simulink model "STM32_UART_Receiver2_2016b"  (R2016b)
settings: Solver=FixedStepDiscrete  StartTime=0.0  StopTime=inf  FixedStep=0.02  RelTol=1e-3  EnableMultiTasking=on
undefined symbols (not defined in the file or in its folder): serial
libraries: xpcutilitieslib x25, etargetslib x25, instrumentlib x2, aerolibanimutils x1
settings Model: Creator=Administrator  LastModifiedBy=Administrator
settings DataIOCC: LimitDataPoints=on  SaveFormat=Array
settings OptimizationCC: LifeSpan=inf
settings DebuggingCC: SFUnexpectedBacktrackingDiag=warning  SFNoUnconditionalDefaultTransitionDiag=warning  SFExecutionAtInitializationDiag=none
settings HardwareCC: ProdBitPerPointer=32  ProdBitPerSizeT=32  ProdBitPerPtrDiffT=32  ProdLargestAtomicFloat=None  ProdIntDivRoundTo=Undefined  ProdEndianess=Unspecified  ProdWordSize=32  ProdHWDeviceType=32-bit Generic
settings ModelReferenceCC: PropagateSignalLabelsOutOfModel=off
settings GRTTargetCC: TargetLangStandard=C89/C90 (ANSI)  GeneratePreprocessorConditionals=Disable all
settings ConfigComp: CovMetricSettings=dw  CovHtmlReporting=on  CovSaveCumulativeToWorkspaceVar=on  CovSaveSingleToWorkspaceVar=on  CovExternalEMLEnable=off

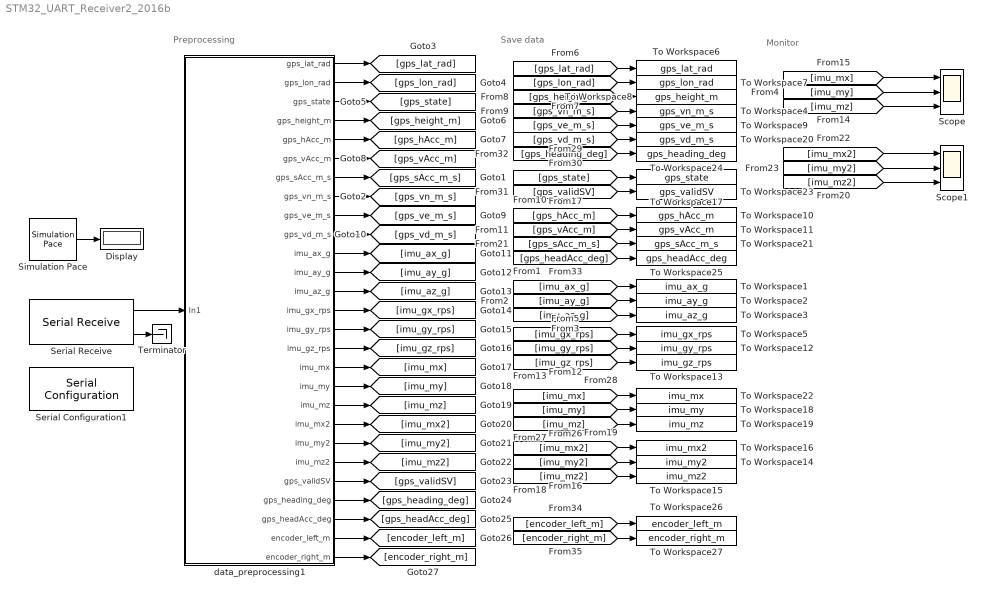
== system STM32_UART_Receiver2_2016b ==
  note: Monitor
  note: Preprocessing
  note: Save data
  Display : Display
  Scope : Scope  NumInputPorts=3
  Scope1 : Scope  NumInputPorts=3
  Serial Configuration1 : instrumentlib/Serial Configuration  Priority=-200000  ComPortMenu=<Please select a port...>  ComPort=COM8  ObjConstructor=serial('COM8');  BaudRate=9600  DataBits=8  Parity=none  StopBits=1  FlowControl=none  Timeout=10  ByteOrder=LittleEndian
  Serial Receive : instrumentlib/Serial Receive  ComPortMenu=<Please select a port...>  ComPort=COM8  ObjConstructor=serial('COM8');  Header=AA1  Terminator=<none>  DataSize="[1  72]"  DataType=uint8  EnableBlockingMode=off  ActionDataUnavailable=Output last received value  CustomValue=0  SampleTime=0.02
  Simulation Pace : aerolibanimutils/Simulation Pace  SimulationPace=1  SleepMode=MATLAB Thread  OutputPaceError=on  SampleTime=0.02
  Terminator : Terminator
  To Workspace1 : ToWorkspace  VariableName=imu_ax_g  SampleTime=-1
      settings: Save2DSignal=2-D array (concatenate along first dimension)
  To Workspace10 : ToWorkspace  VariableName=gps_hAcc_m  SampleTime=-1
      settings: Save2DSignal=2-D array (concatenate along first dimension)
  To Workspace11 : ToWorkspace  VariableName=gps_vAcc_m  SampleTime=-1
      settings: Save2DSignal=2-D array (concatenate along first dimension)
  To Workspace12 : ToWorkspace  VariableName=imu_gy_rps  SampleTime=-1
      settings: Save2DSignal=2-D array (concatenate along first dimension)
  To Workspace13 : ToWorkspace  VariableName=imu_gz_rps  SampleTime=-1
      settings: Save2DSignal=2-D array (concatenate along first dimension)
  To Workspace14 : ToWorkspace  VariableName=imu_my2  SampleTime=-1
      settings: Save2DSignal=2-D array (concatenate along first dimension)
  To Workspace15 : ToWorkspace  VariableName=imu_mz2  SampleTime=-1
      settings: Save2DSignal=2-D array (concatenate along first dimension)
  To Workspace16 : ToWorkspace  VariableName=imu_mx2  SampleTime=-1
      settings: Save2DSignal=2-D array (concatenate along first dimension)
  To Workspace17 : ToWorkspace  VariableName=gps_state  SampleTime=-1
      settings: Save2DSignal=2-D array (concatenate along first dimension)
  To Workspace18 : ToWorkspace  VariableName=imu_my  SampleTime=-1
      settings: Save2DSignal=2-D array (concatenate along first dimension)
  To Workspace19 : ToWorkspace  VariableName=imu_mz  SampleTime=-1
      settings: Save2DSignal=2-D array (concatenate along first dimension)
  To Workspace2 : ToWorkspace  VariableName=imu_ay_g  SampleTime=-1
      settings: Save2DSignal=2-D array (concatenate along first dimension)
  To Workspace20 : ToWorkspace  VariableName=gps_vd_m_s  SampleTime=-1
      settings: Save2DSignal=2-D array (concatenate along first dimension)
  To Workspace21 : ToWorkspace  VariableName=gps_sAcc_m_s  SampleTime=-1
      settings: Save2DSignal=2-D array (concatenate along first dimension)
  To Workspace22 : ToWorkspace  VariableName=imu_mx  SampleTime=-1
      settings: Save2DSignal=2-D array (concatenate along first dimension)
  To Workspace23 : ToWorkspace  VariableName=gps_validSV  SampleTime=-1
      settings: Save2DSignal=2-D array (concatenate along first dimension)
  To Workspace24 : ToWorkspace  VariableName=gps_heading_deg  SampleTime=-1
      settings: Save2DSignal=2-D array (concatenate along first dimension)
  To Workspace25 : ToWorkspace  VariableName=gps_headAcc_deg  SampleTime=-1
      settings: Save2DSignal=2-D array (concatenate along first dimension)
  To Workspace26 : ToWorkspace  VariableName=encoder_left_m  SampleTime=-1
      settings: Save2DSignal=2-D array (concatenate along first dimension)
  To Workspace27 : ToWorkspace  VariableName=encoder_right_m  SampleTime=-1
      settings: Save2DSignal=2-D array (concatenate along first dimension)
  To Workspace3 : ToWorkspace  VariableName=imu_az_g  SampleTime=-1
      settings: Save2DSignal=2-D array (concatenate along first dimension)
  To Workspace4 : ToWorkspace  VariableName=gps_vn_m_s  SampleTime=-1
      settings: Save2DSignal=2-D array (concatenate along first dimension)
  To Workspace5 : ToWorkspace  VariableName=imu_gx_rps  SampleTime=-1
      settings: Save2DSignal=2-D array (concatenate along first dimension)
  To Workspace6 : ToWorkspace  VariableName=gps_lat_rad  SampleTime=-1
      settings: Save2DSignal=2-D array (concatenate along first dimension)
  To Workspace7 : ToWorkspace  VariableName=gps_lon_rad  SampleTime=-1
      settings: Save2DSignal=2-D array (concatenate along first dimension)
  To Workspace8 : ToWorkspace  VariableName=gps_height_m  SampleTime=-1
      settings: Save2DSignal=2-D array (concatenate along first dimension)
  To Workspace9 : ToWorkspace  VariableName=gps_ve_m_s  SampleTime=-1
      settings: Save2DSignal=2-D array (concatenate along first dimension)
  data_preprocessing1 : Subsystem
  wires:
  [gps_lat_rad] -> To Workspace6/1
  [gps_lon_rad] -> To Workspace7/1
  [gps_height_m] -> To Workspace8/1
  [gps_hAcc_m] -> To Workspace10/1
  [gps_vAcc_m] -> To Workspace11/1
  [gps_sAcc_m_s] -> To Workspace21/1
  [imu_ax_g] -> To Workspace1/1
  [imu_ay_g] -> To Workspace2/1
  [imu_az_g] -> To Workspace3/1
  [imu_gx_rps] -> To Workspace5/1
  [imu_gy_rps] -> To Workspace12/1
  [imu_gz_rps] -> To Workspace13/1
  data_preprocessing1/1(gps_lat_rad) -> [gps_lat_rad]
  data_preprocessing1/2(gps_lon_rad) -> [gps_lon_rad]
  data_preprocessing1/3(gps_state) -> [gps_state]
  data_preprocessing1/4(gps_height_m) -> [gps_height_m]
  data_preprocessing1/5(gps_hAcc_m) -> [gps_hAcc_m]
  data_preprocessing1/6(gps_vAcc_m) -> [gps_vAcc_m]
  data_preprocessing1/7(gps_sAcc_m_s) -> [gps_sAcc_m_s]
  data_preprocessing1/8(gps_vn_m_s) -> [gps_vn_m_s]
  data_preprocessing1/9(gps_ve_m_s) -> [gps_ve_m_s]
  data_preprocessing1/10(gps_vd_m_s) -> [gps_vd_m_s]
  data_preprocessing1/11(imu_ax_g) -> [imu_ax_g]
  data_preprocessing1/12(imu_ay_g) -> [imu_ay_g]
  data_preprocessing1/13(imu_az_g) -> [imu_az_g]
  data_preprocessing1/14(imu_gx_rps) -> [imu_gx_rps]
  data_preprocessing1/15(imu_gy_rps) -> [imu_gy_rps]
  data_preprocessing1/16(imu_gz_rps) -> [imu_gz_rps]
  data_preprocessing1/17(imu_mx) -> [imu_mx]
  data_preprocessing1/19(imu_mz) -> [imu_mz]
  [imu_mx] -> To Workspace22/1
  [imu_my] -> To Workspace18/1
  [imu_mz] -> To Workspace19/1
  [gps_state] -> To Workspace17/1
  [gps_vn_m_s] -> To Workspace4/1
  [gps_ve_m_s] -> To Workspace9/1
  [gps_vd_m_s] -> To Workspace20/1
  data_preprocessing1/18(imu_my) -> [imu_my]
  data_preprocessing1/23(gps_validSV) -> [gps_validSV]
  data_preprocessing1/24(gps_heading_deg) -> [gps_heading_deg]
  data_preprocessing1/25(gps_headAcc_deg) -> [gps_headAcc_deg]
  [gps_heading_deg] -> To Workspace24/1
  [gps_headAcc_deg] -> To Workspace25/1
  [gps_validSV] -> To Workspace23/1
  data_preprocessing1/26(encoder_left_m) -> [encoder_left_m]
  data_preprocessing1/27(encoder_right_m) -> [encoder_right_m]
  [encoder_left_m] -> To Workspace26/1
  [encoder_right_m] -> To Workspace27/1
  Serial Receive/1 -> data_preprocessing1/1(In1)
  Simulation Pace/1 -> Display/1
  [imu_mx] -> Scope/1
  [imu_my] -> Scope/2
  [imu_mz] -> Scope/3
  data_preprocessing1/20(imu_mx2) -> [imu_mx2]
  data_preprocessing1/21(imu_my2) -> [imu_my2]
  data_preprocessing1/22(imu_mz2) -> [imu_mz2]
  [imu_mx2] -> To Workspace16/1
  [imu_my2] -> To Workspace14/1
  [imu_mz2] -> To Workspace15/1
  [imu_mx2] -> Scope1/1
  [imu_my2] -> Scope1/2
  [imu_mz2] -> Scope1/3
  Serial Receive/2 -> Terminator/1

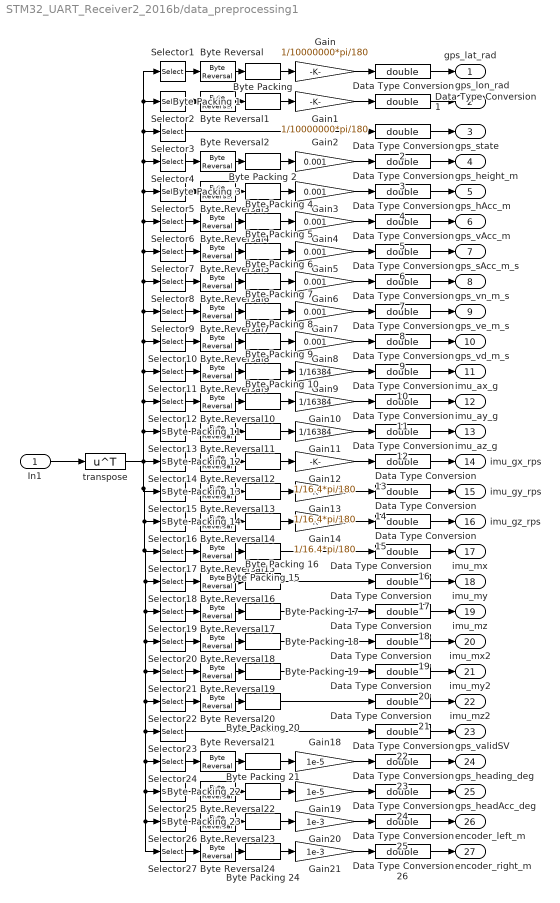
== system STM32_UART_Receiver2_2016b/data_preprocessing1 ==
  In1 : Inport
  Byte Packing {,1..24} (25 alike) : xpcutilitieslib/Byte Packing 
  Byte Reversal{,1..24} (25 alike) : etargetslib/Byte Reversal  numInp=1
  Data Type Conversion{,1..26} (27 alike) : DataTypeConversion  OutDataTypeStr=double
  Gain : Gain  Gain=1/10000000*pi/180
  Gain1 : Gain  Gain=1/10000000*pi/180
  Gain10 : Gain  Gain=1/16384
  Gain11 : Gain  Gain=1/16384
  Gain12 : Gain  Gain=1/16.4*pi/180
  Gain13 : Gain  Gain=1/16.4*pi/180
  Gain14 : Gain  Gain=1/16.4*pi/180
  Gain18 : Gain  Gain=1e-5
  Gain19 : Gain  Gain=1e-5
  Gain{2..8} (7 alike) : Gain  Gain=0.001
  Gain20 : Gain  Gain=1e-3
  Gain21 : Gain  Gain=1e-3
  Gain9 : Gain  Gain=1/16384
  Selector1 : Selector  InputPortWidth=72  IndexOptions=Index vector (dialog)  Indices=[5 4 3 2]  OutputSizes=1
  Selector10 : Selector  InputPortWidth=72  IndexOptions=Index vector (dialog)  Indices=[32 31 30 29]  OutputSizes=1
  Selector11 : Selector  InputPortWidth=72  IndexOptions=Index vector (dialog)  Indices=[34 33]  OutputSizes=1
  Selector12 : Selector  InputPortWidth=72  IndexOptions=Index vector (dialog)  Indices=[36 35]  OutputSizes=1
  Selector13 : Selector  InputPortWidth=72  IndexOptions=Index vector (dialog)  Indices=[38 37]  OutputSizes=1
  Selector14 : Selector  InputPortWidth=72  IndexOptions=Index vector (dialog)  Indices=[40 39]  OutputSizes=1
  Selector15 : Selector  InputPortWidth=72  IndexOptions=Index vector (dialog)  Indices=[42 41]  OutputSizes=1
  Selector16 : Selector  InputPortWidth=72  IndexOptions=Index vector (dialog)  Indices=[44 43]  OutputSizes=1
  Selector17 : Selector  InputPortWidth=72  IndexOptions=Index vector (dialog)  Indices=[46 45]  OutputSizes=1
  Selector18 : Selector  InputPortWidth=72  IndexOptions=Index vector (dialog)  Indices=[48 47]  OutputSizes=1
  Selector19 : Selector  InputPortWidth=72  IndexOptions=Index vector (dialog)  Indices=[50 49]  OutputSizes=1
  Selector2 : Selector  InputPortWidth=72  IndexOptions=Index vector (dialog)  Indices=[9 8 7 6]  OutputSizes=1
  Selector20 : Selector  InputPortWidth=72  IndexOptions=Index vector (dialog)  Indices=[52 51]  OutputSizes=1
  Selector21 : Selector  InputPortWidth=72  IndexOptions=Index vector (dialog)  Indices=[54 53]  OutputSizes=1
  Selector22 : Selector  InputPortWidth=72  IndexOptions=Index vector (dialog)  Indices=[56 55]  OutputSizes=1
  Selector23 : Selector  InputPortWidth=72  IndexOptions=Index vector (dialog)  Indices=57  OutputSizes=1
  Selector24 : Selector  InputPortWidth=72  IndexOptions=Index vector (dialog)  Indices=[61 60 59 58]  OutputSizes=1
  Selector25 : Selector  InputPortWidth=72  IndexOptions=Index vector (dialog)  Indices=[63 62]  OutputSizes=1
  Selector26 : Selector  InputPortWidth=72  IndexOptions=Index vector (dialog)  Indices=[67 66 65 64]  OutputSizes=1
  Selector27 : Selector  InputPortWidth=72  IndexOptions=Index vector (dialog)  Indices=[71 70 69 68]  OutputSizes=1
  Selector3 : Selector  InputPortWidth=72  IndexOptions=Index vector (dialog)  Indices=10  OutputSizes=1
  Selector4 : Selector  InputPortWidth=72  IndexOptions=Index vector (dialog)  Indices=[14 13 12 11]  OutputSizes=1
  Selector5 : Selector  InputPortWidth=72  IndexOptions=Index vector (dialog)  Indices=[16 15]  OutputSizes=1
  Selector6 : Selector  InputPortWidth=72  IndexOptions=Index vector (dialog)  Indices=[18 17]  OutputSizes=1
  Selector7 : Selector  InputPortWidth=72  IndexOptions=Index vector (dialog)  Indices=[20 19]  OutputSizes=1
  Selector8 : Selector  InputPortWidth=72  IndexOptions=Index vector (dialog)  Indices=[24 23 22 21]  OutputSizes=1
  Selector9 : Selector  InputPortWidth=72  IndexOptions=Index vector (dialog)  Indices=[28 27 26 25]  OutputSizes=1
  transpose : Math  Operator=transpose  SaturateOnIntegerOverflow=on
  gps_lat_rad : Outport
  gps_lon_rad : Outport  Port=2
  gps_state : Outport  Port=3
  gps_height_m : Outport  Port=4
  gps_hAcc_m : Outport  Port=5
  gps_vAcc_m : Outport  Port=6
  gps_sAcc_m_s : Outport  Port=7
  gps_vn_m_s : Outport  Port=8
  gps_ve_m_s : Outport  Port=9
  gps_vd_m_s : Outport  Port=10
  imu_ax_g : Outport  Port=11
  imu_ay_g : Outport  Port=12
  imu_az_g : Outport  Port=13
  imu_gx_rps : Outport  Port=14
  imu_gy_rps : Outport  Port=15
  imu_gz_rps : Outport  Port=16
  imu_mx : Outport  Port=17
  imu_my : Outport  Port=18
  imu_mz : Outport  Port=19
  imu_mx2 : Outport  Port=20
  imu_my2 : Outport  Port=21
  imu_mz2 : Outport  Port=22
  gps_validSV : Outport  Port=23
  gps_heading_deg : Outport  Port=24
  gps_headAcc_deg : Outport  Port=25
  encoder_left_m : Outport  Port=26
  encoder_right_m : Outport  Port=27
  wires:
  In1/1 -> transpose/1
  Gain/1 -> Data Type Conversion/1
  "Byte Packing "/1 -> Gain/1
  Selector1/1 -> Byte Reversal/1
  Byte Reversal/1 -> "Byte Packing "/1
  Selector2/1 -> Byte Reversal1/1
  Byte Reversal1/1 -> Byte Packing 1/1
  Byte Packing 1/1 -> Gain1/1
  Gain1/1 -> Data Type Conversion1/1
  Selector3/1 -> Data Type Conversion2/1
  Byte Packing 2/1 -> Gain2/1
  Byte Reversal2/1 -> Byte Packing 2/1
  Selector4/1 -> Byte Reversal2/1
  Gain2/1 -> Data Type Conversion3/1
  Selector5/1 -> Byte Reversal3/1
  Byte Reversal3/1 -> Byte Packing 3/1
  Byte Packing 3/1 -> Gain3/1
  Gain3/1 -> Data Type Conversion4/1
  Selector6/1 -> Byte Reversal4/1
  Byte Reversal4/1 -> Byte Packing 4/1
  Byte Packing 4/1 -> Gain4/1
  Gain4/1 -> Data Type Conversion5/1
  Byte Packing 5/1 -> Gain5/1
  Selector7/1 -> Byte Reversal5/1
  Byte Reversal5/1 -> Byte Packing 5/1
  Gain5/1 -> Data Type Conversion6/1
  Byte Packing 6/1 -> Gain6/1
  Byte Reversal6/1 -> Byte Packing 6/1
  Selector8/1 -> Byte Reversal6/1
  Gain6/1 -> Data Type Conversion7/1
  Byte Reversal7/1 -> Byte Packing 7/1
  Selector9/1 -> Byte Reversal7/1
  Byte Packing 7/1 -> Gain7/1
  Gain7/1 -> Data Type Conversion8/1
  Byte Reversal8/1 -> Byte Packing 8/1
  Selector10/1 -> Byte Reversal8/1
  Byte Packing 8/1 -> Gain8/1
  Gain8/1 -> Data Type Conversion9/1
  Selector11/1 -> Byte Reversal9/1
  Byte Reversal9/1 -> Byte Packing 9/1
  Gain9/1 -> Data Type Conversion10/1
  Byte Packing 9/1 -> Gain9/1
  Byte Reversal10/1 -> Byte Packing 10/1
  Byte Packing 10/1 -> Gain10/1
  Selector12/1 -> Byte Reversal10/1
  Gain10/1 -> Data Type Conversion11/1
  Byte Reversal11/1 -> Byte Packing 11/1
  Selector13/1 -> Byte Reversal11/1
  Byte Packing 11/1 -> Gain11/1
  Gain11/1 -> Data Type Conversion12/1
  Byte Reversal12/1 -> Byte Packing 12/1
  Byte Packing 12/1 -> Gain12/1
  Selector14/1 -> Byte Reversal12/1
  Gain12/1 -> Data Type Conversion13/1
  Byte Packing 13/1 -> Gain13/1
  Byte Reversal13/1 -> Byte Packing 13/1
  Selector15/1 -> Byte Reversal13/1
  Gain13/1 -> Data Type Conversion14/1
  Byte Packing 14/1 -> Gain14/1
  Byte Reversal14/1 -> Byte Packing 14/1
  Selector16/1 -> Byte Reversal14/1
  Gain14/1 -> Data Type Conversion15/1
  Byte Packing 15/1 -> Data Type Conversion16/1
  Selector17/1 -> Byte Reversal15/1
  Byte Reversal15/1 -> Byte Packing 15/1
  Byte Reversal16/1 -> Byte Packing 16/1
  Selector18/1 -> Byte Reversal16/1
  Byte Packing 16/1 -> Data Type Conversion17/1
  Byte Reversal17/1 -> Byte Packing 17/1
  transpose/1 -> Selector27/1, Selector26/1, Selector25/1, Selector24/1, Selector23/1, Selector22/1, Selector21/1, Selector20/1, Selector19/1, Selector18/1, Selector17/1, Selector16/1, Selector15/1, Selector14/1, Selector13/1, Selector12/1, Selector11/1, Selector10/1, Selector9/1, Selector8/1, Selector7/1, Selector6/1, Selector5/1, Selector4/1, Selector3/1, Selector2/1, Selector1/1
  Selector19/1 -> Byte Reversal17/1
  Byte Packing 17/1 -> Data Type Conversion18/1
  Selector20/1 -> Byte Reversal18/1
  Selector21/1 -> Byte Reversal19/1
  Selector22/1 -> Byte Reversal20/1
  Selector24/1 -> Byte Reversal21/1
  Byte Reversal21/1 -> Byte Packing 21/1
  Byte Packing 21/1 -> Gain18/1
  Gain18/1 -> Data Type Conversion23/1
  Byte Packing 22/1 -> Gain19/1
  Byte Reversal22/1 -> Byte Packing 22/1
  Selector25/1 -> Byte Reversal22/1
  Gain19/1 -> Data Type Conversion24/1
  Byte Packing 23/1 -> Gain20/1
  Byte Reversal23/1 -> Byte Packing 23/1
  Selector26/1 -> Byte Reversal23/1
  Gain20/1 -> Data Type Conversion25/1
  Byte Packing 24/1 -> Gain21/1
  Byte Reversal24/1 -> Byte Packing 24/1
  Selector27/1 -> Byte Reversal24/1
  Gain21/1 -> Data Type Conversion26/1
  Selector23/1 -> Data Type Conversion22/1
  Data Type Conversion/1 -> gps_lat_rad/1
  Data Type Conversion1/1 -> gps_lon_rad/1
  Data Type Conversion2/1 -> gps_state/1
  Data Type Conversion3/1 -> gps_height_m/1
  Data Type Conversion4/1 -> gps_hAcc_m/1
  Data Type Conversion5/1 -> gps_vAcc_m/1
  Data Type Conversion6/1 -> gps_sAcc_m_s/1
  Data Type Conversion7/1 -> gps_vn_m_s/1
  Data Type Conversion8/1 -> gps_ve_m_s/1
  Data Type Conversion9/1 -> gps_vd_m_s/1
  Data Type Conversion10/1 -> imu_ax_g/1
  Data Type Conversion11/1 -> imu_ay_g/1
  Data Type Conversion12/1 -> imu_az_g/1
  Data Type Conversion13/1 -> imu_gx_rps/1
  Data Type Conversion14/1 -> imu_gy_rps/1
  Data Type Conversion15/1 -> imu_gz_rps/1
  Data Type Conversion16/1 -> imu_mx/1
  Data Type Conversion17/1 -> imu_my/1
  Data Type Conversion18/1 -> imu_mz/1
  Data Type Conversion22/1 -> gps_validSV/1
  Data Type Conversion23/1 -> gps_heading_deg/1
  Data Type Conversion24/1 -> gps_headAcc_deg/1
  Data Type Conversion25/1 -> encoder_left_m/1
  Data Type Conversion26/1 -> encoder_right_m/1
  Byte Packing 18/1 -> Data Type Conversion19/1
  Byte Reversal18/1 -> Byte Packing 18/1
  Byte Reversal19/1 -> Byte Packing 19/1
  Byte Packing 19/1 -> Data Type Conversion20/1
  Byte Reversal20/1 -> Byte Packing 20/1
  Byte Packing 20/1 -> Data Type Conversion21/1
  Data Type Conversion19/1 -> imu_mx2/1
  Data Type Conversion20/1 -> imu_my2/1
  Data Type Conversion21/1 -> imu_mz2/1
